simulink model "ppi"  (R2020b)
settings: Solver=ode4  StartTime=0.0  StopTime=10.0  FixedStep=0.01  RelTol=1e-3
values from neighbouring files (symbols this model uses):
  dc = [-0.75;3.75]    [script.m]
  get_C = matlabFunction(C)    [script.m]
  get_G = matlabFunction(G)    [script.m]
  get_inv_M = matlabFunction(inv_M)    [script.m]
  get_M = matlabFunction(M)    [script.m]
  Ka = M_bar    [script.m]    (also in test.m = diag([ka1, ka2]))
  Kd = first_order*M_bar    [script.m]    (also in test.m = diag([kd1, kd2]))
  Ki = zero_order*M_bar    [script.m]    (also in test.m = diag([ki1, ki2]))
  Kp = diag([5.67 5.67])    [script.m]    (also in test.m = diag([kp1, kp2]))
  omega = omegas(:,test)    [script.m]
  theta0 = zeros(n_links, 1)    [script.m]
  theta_dot0 = zeros(n_links,1)    [script.m]
settings Model: Creator=lucas  LastModifiedBy=lucas

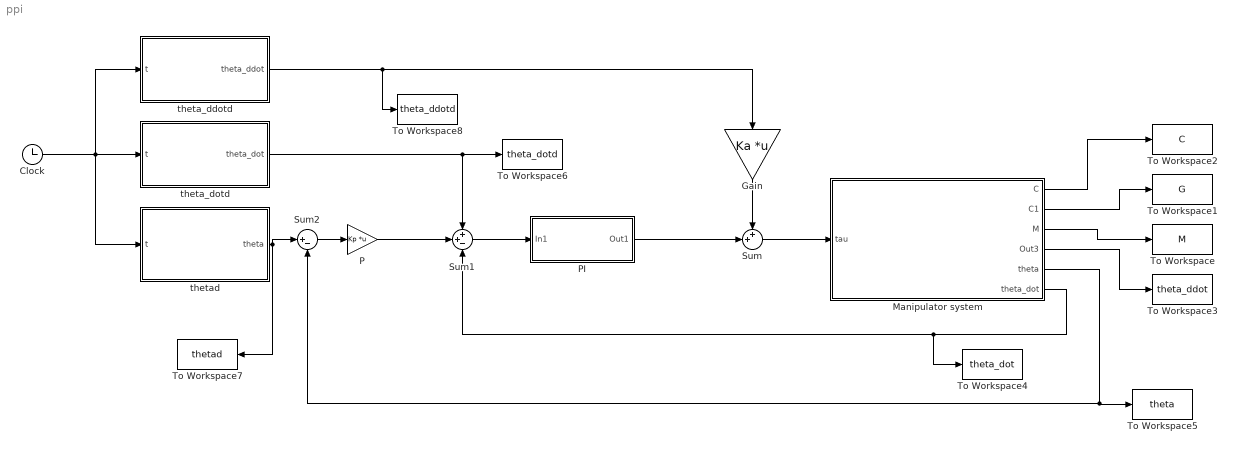
== system ppi ==
  Clock : Clock
  Gain : Gain  Gain=Ka  Multiplication=Matrix(K*u) (u vector)
  Manipulator system : Subsystem
  P : Gain  Gain=Kp  Multiplication=Matrix(K*u) (u vector)
  PI : Subsystem
  Sum : Sum  Inputs=++|
  Sum1 : Sum  Inputs=++-
  Sum2 : Sum  Inputs=|+-
  To Workspace : ToWorkspace  VariableName=M  SaveFormat=Timeseries  SampleTime=-1
  To Workspace1 : ToWorkspace  VariableName=G  SaveFormat=Timeseries  SampleTime=-1
  To Workspace2 : ToWorkspace  VariableName=C  SaveFormat=Timeseries  SampleTime=-1
  To Workspace3 : ToWorkspace  VariableName=theta_ddot  SaveFormat=Timeseries  SampleTime=-1
  To Workspace4 : ToWorkspace  VariableName=theta_dot  SaveFormat=Timeseries  SampleTime=-1
  To Workspace5 : ToWorkspace  VariableName=theta  SaveFormat=Timeseries  SampleTime=-1
  To Workspace6 : ToWorkspace  VariableName=theta_dotd  SaveFormat=Timeseries  SampleTime=-1
  To Workspace7 : ToWorkspace  VariableName=thetad  SaveFormat=Timeseries  SampleTime=-1
  To Workspace8 : ToWorkspace  VariableName=theta_ddotd  SaveFormat=Timeseries  SampleTime=-1
  theta_ddotd : MATLAB Function  TreatAsAtomicUnit=on
  theta_dotd : MATLAB Function  TreatAsAtomicUnit=on
  thetad : MATLAB Function  TreatAsAtomicUnit=on
  wires:
  Clock/1 -> theta_ddotd/1(t), theta_dotd/1(t), thetad/1(t)
  Sum/1 -> Manipulator system/1(tau)
  Gain/1 -> Sum/1
  theta_ddotd/1(theta_ddot) -> To Workspace8/1, Gain/1
  PI/1(Out1) -> Sum/2
  Sum1/1 -> PI/1(In1)
  Manipulator system/6(theta_dot) -> To Workspace4/1, Sum1/3
  Manipulator system/5(theta) -> Sum2/2, To Workspace5/1
  Manipulator system/4(Out3) -> To Workspace3/1
  Manipulator system/1(C) -> To Workspace2/1
  Manipulator system/2(C1) -> To Workspace1/1
  Manipulator system/3(M) -> To Workspace/1
  P/1 -> Sum1/2
  Sum2/1 -> P/1
  thetad/1(theta) -> Sum2/1, To Workspace7/1
  theta_dotd/1(theta_dot) -> Sum1/1, To Workspace6/1

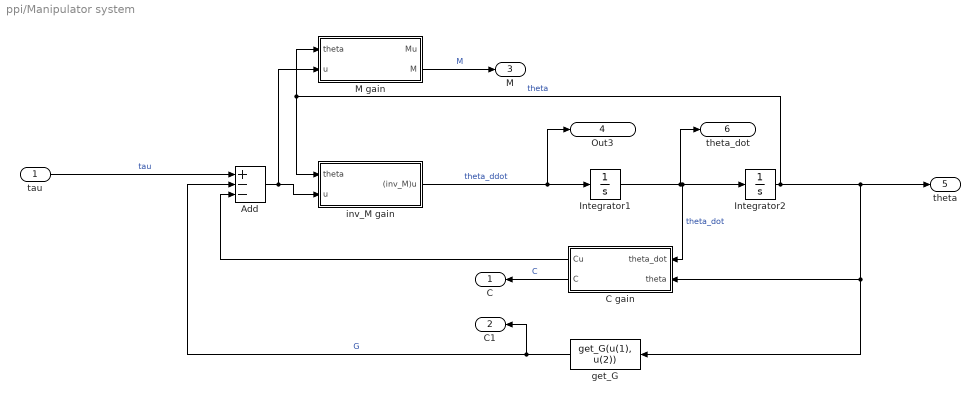
== system ppi/Manipulator system ==
  tau : Inport
  Add : Sum  Inputs=+--
  C gain : Subsystem
  Integrator1 : Integrator  InitialCondition=theta_dot0
  Integrator2 : Integrator  InitialCondition=theta0
  M gain : Subsystem
  get_G : MATLABFcn  MATLABFcn=get_G(u(1), u(2))  Output1D=off
  inv_M gain : Subsystem
  C : Outport
  C1 : Outport  Port=2
  M : Outport  Port=3
  Out3 : Outport  Port=4
  theta : Outport  Port=5
  theta_dot : Outport  Port=6
  wires:
  inv_M gain/1((inv_M)u) -> Integrator1/1, Out3/1  "theta_ddot"
  Integrator1/1 -> C gain/1(theta_dot), Integrator2/1, theta_dot/1  "theta_dot"
  tau/1 -> Add/1  "tau"
  Integrator2/1 -> inv_M gain/1(theta), M gain/1(theta), get_G/1, C gain/2(theta), theta/1  "theta"
  C gain/1(Cu) -> Add/3
  get_G/1 -> C1/1, Add/2  "G"
  Add/1 -> M gain/2(u), inv_M gain/2(u)
  C gain/2(C) -> C/1  "C"
  M gain/2(M) -> M/1  "M"

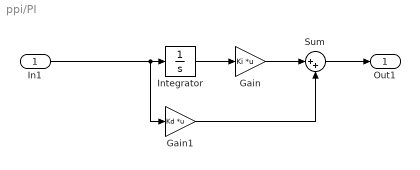
== system ppi/PI ==
  In1 : Inport
  Gain : Gain  Gain=Ki  Multiplication=Matrix(K*u) (u vector)
  Gain1 : Gain  Gain=Kd  Multiplication=Matrix(K*u) (u vector)
  Integrator : Integrator
  Sum : Sum  Inputs=|++
  Out1 : Outport
  wires:
  Integrator/1 -> Gain/1
  In1/1 -> Gain1/1, Integrator/1
  Gain/1 -> Sum/1
  Sum/1 -> Out1/1
  Gain1/1 -> Sum/2

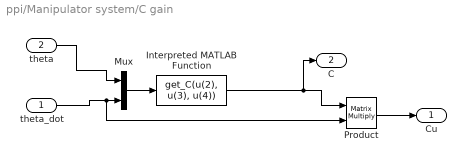
== system ppi/Manipulator system/C gain ==
  theta_dot : Inport
  theta : Inport  Port=2
  Interpreted MATLAB Function : MATLABFcn  MATLABFcn=get_C(u(2), u(3), u(4))  Output1D=off
  Mux : Mux  Inputs=2
  Product : Product  Multiplication=Matrix(*)
  Cu : Outport
  C : Outport  Port=2
  wires:
  Product/1 -> Cu/1
  Interpreted MATLAB Function/1 -> C/1, Product/1
  Mux/1 -> Interpreted MATLAB Function/1
  theta/1 -> Mux/1
  theta_dot/1 -> Product/2, Mux/2

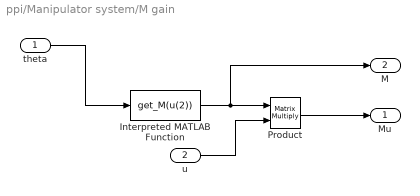
== system ppi/Manipulator system/M gain ==
  theta : Inport
  u : Inport  Port=2
  Interpreted MATLAB Function : MATLABFcn  MATLABFcn=get_M(u(2))  Output1D=off
  Product : Product  Multiplication=Matrix(*)
  Mu : Outport
  M : Outport  Port=2
  wires:
  Product/1 -> Mu/1
  Interpreted MATLAB Function/1 -> M/1, Product/1
  u/1 -> Product/2
  theta/1 -> Interpreted MATLAB Function/1

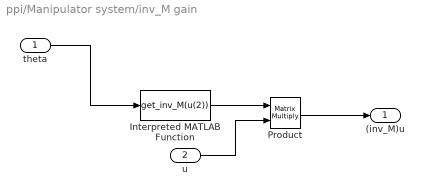
== system ppi/Manipulator system/inv_M gain ==
  theta : Inport
  u : Inport  Port=2
  Interpreted MATLAB Function : MATLABFcn  MATLABFcn=get_inv_M(u(2))  Output1D=off
  Product : Product  Multiplication=Matrix(*)
  (inv_M)u : Outport
  wires:
  Product/1 -> (inv_M)u/1
  Interpreted MATLAB Function/1 -> Product/1
  theta/1 -> Interpreted MATLAB Function/1
  u/1 -> Product/2

== matlab function ppi/thetad ==
  data: t input; theta output; omega parameter; dc parameter
function theta = trajectory(t, omega, dc)
    n = length(omega);
    theta = zeros(n,1);
    for i=1:n
        theta(i) = -0.75*cos(omega(i)*t) + dc(i);
    end

== matlab function ppi/theta_ddotd ==
  data: t input; theta_ddot output; omega parameter
function theta_ddot = accel(t, omega)
    n = length(omega);
    theta_ddot = zeros(n,1);
    for i=1:n
        theta_ddot(i) = 0.75*(omega(i)^2)*cos(omega(i)*t);
    end

== matlab function ppi/theta_dotd ==
  data: t input; theta_dot output; omega parameter
function theta_dot = velocity(t, omega)
    n = length(omega);
    theta_dot = zeros(n,1);
    for i=1:n
        theta_dot(i) = 0.75*omega(i)*sin(omega(i)*t);
    end
